simulink model "modeltask5"  (R2023b)
settings: Solver=VariableStepAuto  StartTime=0.0  StopTime=20  RelTol=1e-3
values from neighbouring files (symbols this model uses):
  A = [0,mf*g*h/Jconst,0,-mf*g/Jconst; 1,0,0,0; 0,-g,0,0; 0,0,1,0]    [task5.m]
  B = [1/Jconst;0;0;0]    [task5.m]
  kT_pi = kpi(1:4)-P*C    [task5.m]
  P = 1/(C*inv(B*kT-A)*B)    [task5.m]
  PI = -kpi(5)    [task5.m]
settings Model: Creator=Krish  LastModifiedBy=Krish

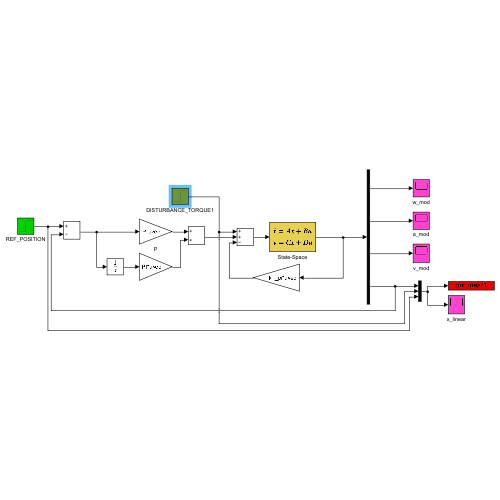
[thumbnail: Simulink's stored preview of the top-level diagram]
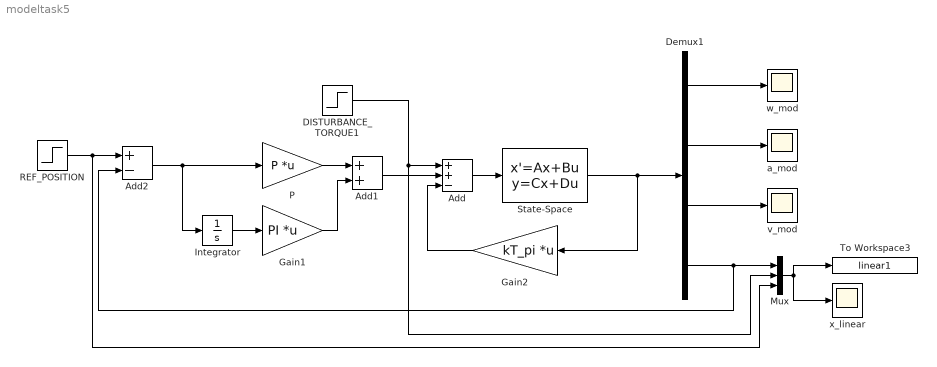
== system modeltask5 ==
  Add : Sum  Inputs=++-
  Add1 : Sum
  Add2 : Sum  Inputs=+-
  DISTURBANCE_TORQUE1 : Step  Time=15  After=0.1  SampleTime=0
  Demux1 : Demux
  Gain1 : Gain  Gain=PI  Multiplication=Matrix(K*u) (u vector)
  Gain2 : Gain  Gain=kT_pi  Multiplication=Matrix(K*u) (u vector)
  Integrator : Integrator
  Mux : Mux  Inputs=3
  P : Gain  Gain=P  Multiplication=Matrix(K*u) (u vector)
  REF_POSITION : Step  SampleTime=0
  State-Space : StateSpace  A=A  B=B  C=eye(4)  D=[0;0;0;0]  InitialCondition=0
  To Workspace3 : ToWorkspace  VariableName=linear1  SaveFormat=Timeseries  SampleTime=-1
  a_mod : Scope
  v_mod : Scope
  w_mod : Scope
  x_linear : Scope
  wires:
  Demux1/3 -> v_mod/1
  Demux1/1 -> w_mod/1
  Demux1/2 -> a_mod/1
  Demux1/4 -> Add2/2, Mux/1
  Mux/1 -> x_linear/1, To Workspace3/1
  State-Space/1 -> Gain2/1, Demux1/1
  Gain2/1 -> Add/3
  Add/1 -> State-Space/1
  DISTURBANCE_TORQUE1/1 -> Mux/2, Add/1
  Add1/1 -> Add/2
  P/1 -> Add1/1
  REF_POSITION/1 -> Mux/3, Add2/1
  Add2/1 -> Integrator/1, P/1
  Integrator/1 -> Gain1/1
  Gain1/1 -> Add1/2
